simulink subsystem "Guidance_Team2"  (R2022b)
settings: Solver=VariableStepAuto  StartTime=0.0  StopTime=10.0  RelTol=1e-3
settings Model: Creator=Sahil Gaurkar  LastModifiedBy=Sahil Gaurkar

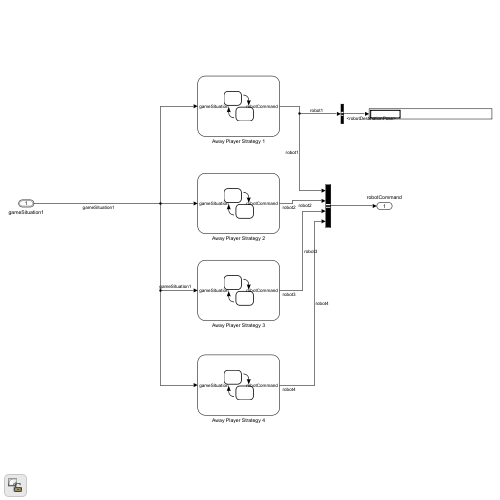
[thumbnail: Simulink's stored preview of the top-level diagram]
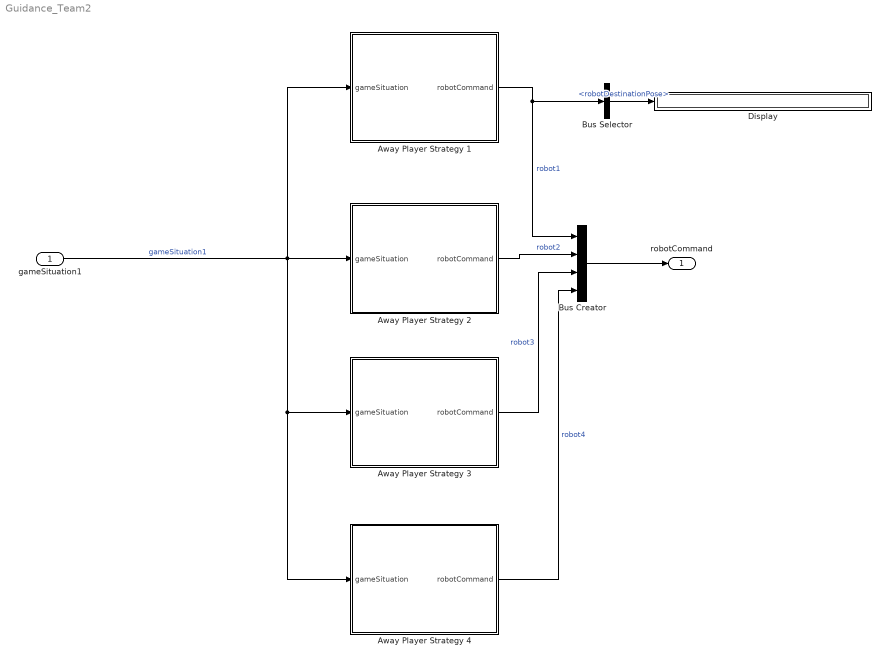
== system Guidance_Team2 ==
  gameSituation1 : Inport  OutDataTypeStr=Bus: gameSituation
  Away Player Strategy 1 : Stateflow chart  TreatAsAtomicUnit=on
  Away Player Strategy 2 : Stateflow chart  TreatAsAtomicUnit=on
  Away Player Strategy 3 : Stateflow chart  TreatAsAtomicUnit=on
  Away Player Strategy 4 : Stateflow chart  TreatAsAtomicUnit=on
  Bus Creator : BusCreator  Inputs=4
  Bus Selector : BusSelector  OutputSignals=robotDestinationPose
  Display : Display
  robotCommand : Outport
  wires:
  Away Player Strategy 3/1(robotCommand) -> Bus Creator/3  "robot3"
  gameSituation1/1 -> Away Player Strategy 3/1(gameSituation), Away Player Strategy 4/1(gameSituation), Away Player Strategy 1/1(gameSituation), Away Player Strategy 2/1(gameSituation)  "gameSituation1"
  Away Player Strategy 2/1(robotCommand) -> Bus Creator/2  "robot2"
  Bus Selector/1 -> Display/1  "<robotDestinationPose>"
  Away Player Strategy 4/1(robotCommand) -> Bus Creator/4  "robot4"
  Away Player Strategy 1/1(robotCommand) -> Bus Selector/1, Bus Creator/1  "robot1"
  Bus Creator/1 -> robotCommand/1

== stateflow chart Guidance_Team2/Away Player Strategy 1 ==
  state InitialState
    en,du:
    if gameSituation.kickConfirmation == true
    robotCommand.kick = false;
    end
    id = 1; % Team1(Home) Robot 1
    shootDistThres = 2500;
    kickableAreaRadius = 20;
    homeGoalPose = [5000, 0];
    awayGoalPose = [-5000, 0];
    homeAttackPositions = [[-3500, 0, 180]; [-2500, 1500, 180]; [-2500, -1500, 180]; [2500, 0, 180]];
    homeDefendPositions = [[1000, 0, 180]; [3000, 1500, 180]; [3000, -1500, 180]; [4000, 0, 180]];
  state ROBOT 1 [group]
    (Strategy for robot 1~3)
  state Attack
    en,du:
    %%calculate the distance to the goal
    teamDistToGoal = [0 0 0 0];
    for idx=1:1:4
    teamDistToGoal(idx) = distTo(gameSituation.robotCurrentPose(idx,1:2), awayGoalPose);
    end
    distToGoal1 = distTo(gameSituation.robotCurrentPose(id,1:2), awayGoalPose);
    %calculate the distance to the ball
    teamDistToBall = [0 0 0 0];
    for idx=1:1:4
    teamDistToBall(idx) = distTo(gameSituation.robotCurrentPose(idx,1:2), ...
    gameSituation.ballCurrentPose(1:2));
    end
    distToBall = distTo(gameSituation.robotCurrentPose(id,1:2), ...
    gameSituation.ballCurrentPose(1:2));
  state Defend
    en,du:
    %%calculate the distance to the home goal
    teamDistToOwnGoal = [0 0 0 0];
    for idx=1:1:4
    teamDistToOwnGoal(idx) = distTo(gameSituation.robotCurrentPose(idx,1:2), homeGoalPose);
    end
    distToOwnGoal = distTo(gameSituation.robotCurrentPose(id,1:2), homeGoalPose);
    for idx=1:1:4
    teamDistToBall(idx) = distTo(gameSituation.robotCurrentPose(idx,1:2), ...
    gameSituation.ballCurrentPose(1:2));
    end
    distToBall = distTo(gameSituation.robotCurrentPose(id,1:2), ...
    gameSituation.ballCurrentPose(1:2));
  state Position
    en,du:
    playerAttackPosition = homeAttackPositions(id, :);
    kickPower = 1;
    kickState = false;
    desiredPosition = playerAttackPosition;
    isdone = true;
  state Shoot
    en,du:
    angleBallGoal = atan2d(awayGoalPose(2) - gameSituation.ballCurrentPose(2), ...
    awayGoalPose(1) - gameSituation.ballCurrentPose(1));
    kickPower = 450;
    kickState = true;
    kickDirection = angleBallGoal;
    xPosition= gameSituation.ballCurrentPose(1) + cosd(180 - angleBallGoal) * kickableAreaRadius;
    yPosition = gameSituation.ballCurrentPose(2) + sind(180 - angleBallGoal) * kickableAreaRadius;
    desiredPosition = [xPosition, yPosition, kickDirection];
    isdone = true;
  state Pass
    en,du:
    [minval,minidx] = min(teamDistToGoal)
    angleBallPlayer = atan2d(gameSituation.robotCurrentPose(minidx, 2) - gameSituation.ballCurrentPose(2), ...
    gameSituation.robotCurrentPose(minidx, 1) - gameSituation.ballCurrentPose(1));
    distBallPlayer = norm(gameSituation.robotCurrentPose(minidx, 1:2) - gameSituation.ballCurrentPose(1:2));
    kickPower = distBallPlayer/4.9;
    kickState = true;
    kickDirection = angleBallPlayer;
    xPosition= gameSituation.ballCurrentPose(1) + cosd(180 - angleBallGoal) * kickableAreaRadius;
    yPosition = gameSituation.ballCurrentPose(2) + sind(180 - angleBallGoal) * kickableAreaRadius;
    desiredPosition = [xPosition, yPosition, kickDirection];
    isdone = true;
  state Dribble
    en,du:
    angleBallGoal = atan2d(awayGoalPose(2) - gameSituation.ballCurrentPose(2), ...
    awayGoalPose(1) - gameSituation.ballCurrentPose(1));
    kickPower = 100;
    %%should be designed as the kickPower = kickPowerCofficent * 100
    %%kickPowerCofficieant should also be calculated by distance
    kickState = true;
    kickDirection = angleBallGoal;
    xPosition= gameSituation.ballCurrentPose(1) + cosd(180 - angleBallGoal) * kickableAreaRadius;
    yPosition = gameSituation.ballCurrentPose(2) + sind(180 - angleBallGoal) * kickableAreaRadius;
    desiredPosition = [xPosition, yPosition, kickDirection];
    isdone = true;
  state Intercept
    en,du:
    angleBallGoal = gameSituation.robotCurrentPose(id, 3);
    kickPower = 150;
    kickState = true;
    kickDirection = angleBallGoal;
    xPosition= gameSituation.ballCurrentPose(1) + cosd(180 - angleBallGoal) * kickableAreaRadius;
    yPosition = gameSituation.ballCurrentPose(2) + sind(180 - angleBallGoal) * kickableAreaRadius;
    desiredPosition = [xPosition, yPosition, kickDirection];
    isdone = true;
  state Formation
    en,du:
    playerDefendPosition = homeDefendPositions(id, :);
    kickPower = 1;
    kickState = false;
    desiredPosition = playerDefendPosition;
    isdone = true;
  state Kick
    state MoveTo1
      en,du:
      isdone = false;
      robotCommand.robotDestinationPose = desiredPosition;
      distToBall = distTo(gameSituation.robotCurrentPose(id,1:2), ...
      gameSituation.ballCurrentPose(1:2));
    state KickTo
      en,du:
      robotCommand.kick = kickState;
      robotCommand.kickProperty = kickPower;
      isdone = true;
    MoveTo1 -> KickTo [order 1] : [distToBall <= kickableAreaRadius+5]
  MoveTo1 -> InitialState [order 2] : [after(1,sec)]
  KickTo -> InitialState : [after(1,sec)]
  (default) -> InitialState
  InitialState -> Attack [order 2] : [gameSituation.ballLastCommandBy(1) == 2]
  InitialState -> Defend [order 1] : [gameSituation.ballLastCommandBy(1) == 1]
  Attack -> Position [order 1] : [distToBall ~= min(teamDistToBall)]
  Defend -> Intercept [order 1] : [distToBall ~= max(teamDistToBall)]
  Defend -> Formation [order 2] : [distToBall == max(teamDistToBall)]
  Attack -> Pass [order 3] : [distToGoal1 ~= min(teamDistToGoal)&& distToBall == min(teamDistToBall)]
  Attack -> Dribble [order 4] : [distToBall == min(teamDistToBall) && distToGoal1 == min(teamDistToGoal) && distToGoal1 > shootDistThres]
  Attack -> Shoot [order 2] : [distToBall == min(teamDistToBall) && distToGoal1 == min(teamDistToGoal) && distToGoal1 < shootDistThres]
  Intercept -> MoveTo1 : [isdone]
  Formation -> MoveTo1 : [isdone]
  Pass -> MoveTo1 : [isdone]
  Dribble -> MoveTo1 : [isdone]
  Shoot -> MoveTo1 : [isdone]
  Position -> MoveTo1 : [isdone]
  data: robotPosition function_input; goalPosition function_input; dist function_output; awayGoalPose local =[0 0]; homeGoalPose local =[0 0]; id local =1; idx local; angleBallGoal local =0; desiredPosition local =[0 0 0]; distToOwnGoal local =0; kickDirection local =0; kickPower local =0; kickState local =false; minidx local; playerDefendPosition local =[0 0 0]; teamDistToGoal local =[0 0 0 0]; teamDistToOwnGoal local =[0 0 0 0]; minval local; isdone local boolean =false; playerAttackPosition local =[0 0 0]; shootDistThres local =0; gameSituation input Bus: gameSituation; kickableAreaRadius local =0; distToGoal1 local =0; angleBallPlayer local =0; robotCommand output Bus: robotCommand; distToBall local =0; teamDistToBall local =[0 0 0 0]; homeAttackPositions local =[0 0 0;0 0 0;0 0 0;0 0 0]; homeDefendPositions local =[0 0 0;0 0 0;0 0 0;0 0 0]; xPosition local; yPosition local; distBallPlayer local
  function dist = distTo(robotPosition,goalPosition):
    | function dist = distTo(robotPosition,goalPosition)
    |     dist = norm(robotPosition - goalPosition);
    | end

== stateflow chart Guidance_Team2/Away Player Strategy 2 ==
  state InitialState
    en,du:
    if gameSituation.kickConfirmation == true
    robotCommand.kick = false;
    end
    id = 2; % Team1(Home) Robot 1
    shootDistThres = 2500;
    kickableAreaRadius = 20;
    homeGoalPose = [5000, 0];
    awayGoalPose = [-5000, 0];
    homeAttackPositions = [[-3500, 0, 180]; [-2500, 1500, 180]; [-2500, -1500, 180]; [2500, 0, 180]];
    homeDefendPositions = [[1000, 0, 180]; [3000, 1500, 180]; [3000, -1500, 180]; [4000, 0, 180]];
  state ROBOT 1 [group]
    (Strategy for robot 1~3)
  state Attack
    en,du:
    %%calculate the distance to the goal
    teamDistToGoal = [0 0 0 0];
    for idx=1:1:4
    teamDistToGoal(idx) = distTo(gameSituation.robotCurrentPose(idx,1:2), awayGoalPose);
    end
    distToGoal1 = distTo(gameSituation.robotCurrentPose(id,1:2), awayGoalPose);
    %calculate the distance to the ball
    teamDistToBall = [0 0 0 0];
    for idx=1:1:4
    teamDistToBall(idx) = distTo(gameSituation.robotCurrentPose(idx,1:2), ...
    gameSituation.ballCurrentPose(1:2));
    end
    distToBall = distTo(gameSituation.robotCurrentPose(id,1:2), ...
    gameSituation.ballCurrentPose(1:2));
  state Defend
    en,du:
    %%calculate the distance to the home goal
    teamDistToOwnGoal = [0 0 0 0];
    for idx=1:1:4
    teamDistToOwnGoal(idx) = distTo(gameSituation.robotCurrentPose(idx,1:2), homeGoalPose);
    end
    distToOwnGoal = distTo(gameSituation.robotCurrentPose(id,1:2), homeGoalPose);
    for idx=1:1:4
    teamDistToBall(idx) = distTo(gameSituation.robotCurrentPose(idx,1:2), ...
    gameSituation.ballCurrentPose(1:2));
    end
    distToBall = distTo(gameSituation.robotCurrentPose(id,1:2), ...
    gameSituation.ballCurrentPose(1:2));
  state Position
    en,du:
    playerAttackPosition = homeAttackPositions(id, :);
    kickPower = 1;
    kickState = false;
    desiredPosition = playerAttackPosition;
    isdone = true;
  state Shoot
    en,du:
    angleBallGoal = atan2d(awayGoalPose(2) - gameSituation.ballCurrentPose(2), ...
    awayGoalPose(1) - gameSituation.ballCurrentPose(1));
    kickPower = 450;
    kickState = true;
    kickDirection = angleBallGoal;
    xPosition= gameSituation.ballCurrentPose(1) + cosd(180 - angleBallGoal) * kickableAreaRadius;
    yPosition = gameSituation.ballCurrentPose(2) + sind(180 - angleBallGoal) * kickableAreaRadius;
    desiredPosition = [xPosition, yPosition, kickDirection];
    isdone = true;
  state Pass
    en,du:
    [minval,minidx] = min(teamDistToGoal)
    angleBallPlayer = atan2d(gameSituation.robotCurrentPose(minidx, 2) - gameSituation.ballCurrentPose(2), ...
    gameSituation.robotCurrentPose(minidx, 1) - gameSituation.ballCurrentPose(1));
    distBallPlayer = norm(gameSituation.robotCurrentPose(minidx, 1:2) - gameSituation.ballCurrentPose(1:2));
    kickPower = distBallPlayer/4.9;
    kickState = true;
    kickDirection = angleBallPlayer;
    xPosition= gameSituation.ballCurrentPose(1) + cosd(180 - angleBallGoal) * kickableAreaRadius;
    yPosition = gameSituation.ballCurrentPose(2) + sind(180 - angleBallGoal) * kickableAreaRadius;
    desiredPosition = [xPosition, yPosition, kickDirection];
    isdone = true;
  state Dribble
    en,du:
    angleBallGoal = atan2d(awayGoalPose(2) - gameSituation.ballCurrentPose(2), ...
    awayGoalPose(1) - gameSituation.ballCurrentPose(1));
    kickPower = 100;
    %%should be designed as the kickPower = kickPowerCofficent * 100
    %%kickPowerCofficieant should also be calculated by distance
    kickState = true;
    kickDirection = angleBallGoal;
    xPosition= gameSituation.ballCurrentPose(1) + cosd(180 - angleBallGoal) * kickableAreaRadius;
    yPosition = gameSituation.ballCurrentPose(2) + sind(180 - angleBallGoal) * kickableAreaRadius;
    desiredPosition = [xPosition, yPosition, kickDirection];
    isdone = true;
  state Intercept
    en,du:
    angleBallGoal = gameSituation.robotCurrentPose(id, 3);
    kickPower = 150;
    kickState = true;
    kickDirection = angleBallGoal;
    xPosition= gameSituation.ballCurrentPose(1) + cosd(180 - angleBallGoal) * kickableAreaRadius;
    yPosition = gameSituation.ballCurrentPose(2) + sind(180 - angleBallGoal) * kickableAreaRadius;
    desiredPosition = [xPosition, yPosition, kickDirection];
    isdone = true;
  state Formation
    en,du:
    playerDefendPosition = homeDefendPositions(id, :);
    kickPower = 1;
    kickState = false;
    desiredPosition = playerDefendPosition;
    isdone = true;
  state Kick
    state MoveTo1
      en,du:
      isdone = false;
      robotCommand.robotDestinationPose = desiredPosition;
      distToBall = distTo(gameSituation.robotCurrentPose(id,1:2), ...
      gameSituation.ballCurrentPose(1:2));
    state KickTo
      en,du:
      robotCommand.kick = kickState;
      robotCommand.kickProperty = kickPower;
      isdone = true;
    MoveTo1 -> KickTo [order 1] : [distToBall <= kickableAreaRadius+5]
  MoveTo1 -> InitialState [order 2] : [after(1,sec)]
  KickTo -> InitialState : [after(1,sec)]
  (default) -> InitialState
  InitialState -> Attack [order 2] : [gameSituation.ballLastCommandBy(1) == 2]
  InitialState -> Defend [order 1] : [gameSituation.ballLastCommandBy(1) == 1]
  Attack -> Position [order 1] : [distToBall ~= min(teamDistToBall)]
  Defend -> Intercept [order 1] : [distToBall ~= max(teamDistToBall)]
  Defend -> Formation [order 2] : [distToBall == max(teamDistToBall)]
  Attack -> Pass [order 3] : [distToGoal1 ~= min(teamDistToGoal)&& distToBall == min(teamDistToBall)]
  Attack -> Dribble [order 4] : [distToBall == min(teamDistToBall) && distToGoal1 == min(teamDistToGoal) && distToGoal1 > shootDistThres]
  Attack -> Shoot [order 2] : [distToBall == min(teamDistToBall) && distToGoal1 == min(teamDistToGoal) && distToGoal1 < shootDistThres]
  Intercept -> MoveTo1 : [isdone]
  Formation -> MoveTo1 : [isdone]
  Pass -> MoveTo1 : [isdone]
  Dribble -> MoveTo1 : [isdone]
  Shoot -> MoveTo1 : [isdone]
  Position -> MoveTo1 : [isdone]
  data: robotPosition function_input; goalPosition function_input; dist function_output; awayGoalPose local =[0 0]; homeGoalPose local =[0 0]; id local =1; idx local; angleBallGoal local =0; desiredPosition local =[0 0 0]; distToOwnGoal local =0; kickDirection local =0; kickPower local =0; kickState local =false; minidx local; playerDefendPosition local =[0 0 0]; teamDistToGoal local =[0 0 0 0]; teamDistToOwnGoal local =[0 0 0 0]; minval local; isdone local boolean =false; playerAttackPosition local =[0 0 0]; shootDistThres local =0; gameSituation input Bus: gameSituation; kickableAreaRadius local =0; distToGoal1 local =0; angleBallPlayer local =0; robotCommand output Bus: robotCommand; distToBall local =0; teamDistToBall local =[0 0 0 0]; homeAttackPositions local =[0 0 0;0 0 0;0 0 0;0 0 0]; homeDefendPositions local =[0 0 0;0 0 0;0 0 0;0 0 0]; xPosition local; yPosition local; distBallPlayer local
  function dist = distTo(robotPosition,goalPosition):
    | function dist = distTo(robotPosition,goalPosition)
    |     dist = norm(robotPosition - goalPosition);
    | end

== stateflow chart Guidance_Team2/Away Player Strategy 3 ==
  state InitialState
    en,du:
    if gameSituation.kickConfirmation == true
    robotCommand.kick = false;
    end
    id = 3; % Team1(Home) Robot 1
    shootDistThres = 2500;
    kickableAreaRadius = 20;
    homeGoalPose = [5000, 0];
    awayGoalPose = [-5000, 0];
    homeAttackPositions = [[-3500, 0, 180]; [-2500, 1500, 180]; [-2500, -1500, 180]; [2500, 0, 180]];
    homeDefendPositions = [[1000, 0, 180]; [3000, 1500, 180]; [3000, -1500, 180]; [4000, 0, 180]];
  state ROBOT 1 [group]
    (Strategy for robot 1~3)
  state Attack
    en,du:
    %%calculate the distance to the goal
    teamDistToGoal = [0 0 0 0];
    for idx=1:1:4
    teamDistToGoal(idx) = distTo(gameSituation.robotCurrentPose(idx,1:2), awayGoalPose);
    end
    distToGoal1 = distTo(gameSituation.robotCurrentPose(id,1:2), awayGoalPose);
    %calculate the distance to the ball
    teamDistToBall = [0 0 0 0];
    for idx=1:1:4
    teamDistToBall(idx) = distTo(gameSituation.robotCurrentPose(idx,1:2), ...
    gameSituation.ballCurrentPose(1:2));
    end
    distToBall = distTo(gameSituation.robotCurrentPose(id,1:2), ...
    gameSituation.ballCurrentPose(1:2));
  state Defend
    en,du:
    %%calculate the distance to the home goal
    teamDistToOwnGoal = [0 0 0 0];
    for idx=1:1:4
    teamDistToOwnGoal(idx) = distTo(gameSituation.robotCurrentPose(idx,1:2), homeGoalPose);
    end
    distToOwnGoal = distTo(gameSituation.robotCurrentPose(id,1:2), homeGoalPose);
    for idx=1:1:4
    teamDistToBall(idx) = distTo(gameSituation.robotCurrentPose(idx,1:2), ...
    gameSituation.ballCurrentPose(1:2));
    end
    distToBall = distTo(gameSituation.robotCurrentPose(id,1:2), ...
    gameSituation.ballCurrentPose(1:2));
  state Position
    en,du:
    playerAttackPosition = homeAttackPositions(id, :);
    kickPower = 1;
    kickState = false;
    desiredPosition = playerAttackPosition;
    isdone = true;
  state Shoot
    en,du:
    angleBallGoal = atan2d(awayGoalPose(2) - gameSituation.ballCurrentPose(2), ...
    awayGoalPose(1) - gameSituation.ballCurrentPose(1));
    kickPower = 450;
    kickState = true;
    kickDirection = angleBallGoal;
    xPosition= gameSituation.ballCurrentPose(1) + cosd(180 - angleBallGoal) * kickableAreaRadius;
    yPosition = gameSituation.ballCurrentPose(2) + sind(180 - angleBallGoal) * kickableAreaRadius;
    desiredPosition = [xPosition, yPosition, kickDirection];
    isdone = true;
  state Pass
    en,du:
    [minval,minidx] = min(teamDistToGoal)
    angleBallPlayer = atan2d(gameSituation.robotCurrentPose(minidx, 2) - gameSituation.ballCurrentPose(2), ...
    gameSituation.robotCurrentPose(minidx, 1) - gameSituation.ballCurrentPose(1));
    distBallPlayer = norm(gameSituation.robotCurrentPose(minidx, 1:2) - gameSituation.ballCurrentPose(1:2));
    kickPower = distBallPlayer/4.9;
    kickState = true;
    kickDirection = angleBallPlayer;
    xPosition= gameSituation.ballCurrentPose(1) + cosd(180 - angleBallGoal) * kickableAreaRadius;
    yPosition = gameSituation.ballCurrentPose(2) + sind(180 - angleBallGoal) * kickableAreaRadius;
    desiredPosition = [xPosition, yPosition, kickDirection];
    isdone = true;
  state Dribble
    en,du:
    angleBallGoal = atan2d(awayGoalPose(2) - gameSituation.ballCurrentPose(2), ...
    awayGoalPose(1) - gameSituation.ballCurrentPose(1));
    kickPower = 100;
    %%should be designed as the kickPower = kickPowerCofficent * 100
    %%kickPowerCofficieant should also be calculated by distance
    kickState = true;
    kickDirection = angleBallGoal;
    xPosition= gameSituation.ballCurrentPose(1) + cosd(180 - angleBallGoal) * kickableAreaRadius;
    yPosition = gameSituation.ballCurrentPose(2) + sind(180 - angleBallGoal) * kickableAreaRadius;
    desiredPosition = [xPosition, yPosition, kickDirection];
    isdone = true;
  state Intercept
    en,du:
    angleBallGoal = gameSituation.robotCurrentPose(id, 3);
    kickPower = 150;
    kickState = true;
    kickDirection = angleBallGoal;
    xPosition= gameSituation.ballCurrentPose(1) + cosd(180 - angleBallGoal) * kickableAreaRadius;
    yPosition = gameSituation.ballCurrentPose(2) + sind(180 - angleBallGoal) * kickableAreaRadius;
    desiredPosition = [xPosition, yPosition, kickDirection];
    isdone = true;
  state Formation
    en,du:
    playerDefendPosition = homeDefendPositions(id, :);
    kickPower = 1;
    kickState = false;
    desiredPosition = playerDefendPosition;
    isdone = true;
  state Kick
    state MoveTo1
      en,du:
      isdone = false;
      robotCommand.robotDestinationPose = desiredPosition;
      distToBall = distTo(gameSituation.robotCurrentPose(id,1:2), ...
      gameSituation.ballCurrentPose(1:2));
    state KickTo
      en,du:
      robotCommand.kick = kickState;
      robotCommand.kickProperty = kickPower;
      isdone = true;
    MoveTo1 -> KickTo [order 1] : [distToBall <= kickableAreaRadius+5]
  MoveTo1 -> InitialState [order 2] : [after(1,sec)]
  KickTo -> InitialState : [after(1,sec)]
  (default) -> InitialState
  InitialState -> Attack [order 2] : [gameSituation.ballLastCommandBy(1) == 2]
  InitialState -> Defend [order 1] : [gameSituation.ballLastCommandBy(1) == 1]
  Attack -> Position [order 1] : [distToBall ~= min(teamDistToBall)]
  Defend -> Intercept [order 1] : [distToBall ~= max(teamDistToBall)]
  Defend -> Formation [order 2] : [distToBall == max(teamDistToBall)]
  Attack -> Pass [order 3] : [distToGoal1 ~= min(teamDistToGoal)&& distToBall == min(teamDistToBall)]
  Attack -> Dribble [order 4] : [distToBall == min(teamDistToBall) && distToGoal1 == min(teamDistToGoal) && distToGoal1 > shootDistThres]
  Attack -> Shoot [order 2] : [distToBall == min(teamDistToBall) && distToGoal1 == min(teamDistToGoal) && distToGoal1 < shootDistThres]
  Intercept -> MoveTo1 : [isdone]
  Formation -> MoveTo1 : [isdone]
  Pass -> MoveTo1 : [isdone]
  Dribble -> MoveTo1 : [isdone]
  Shoot -> MoveTo1 : [isdone]
  Position -> MoveTo1 : [isdone]
  data: robotPosition function_input; goalPosition function_input; dist function_output; awayGoalPose local =[0 0]; homeGoalPose local =[0 0]; id local =1; idx local; angleBallGoal local =0; desiredPosition local =[0 0 0]; distToOwnGoal local =0; kickDirection local =0; kickPower local =0; kickState local =false; minidx local; playerDefendPosition local =[0 0 0]; teamDistToGoal local =[0 0 0 0]; teamDistToOwnGoal local =[0 0 0 0]; minval local; isdone local boolean =false; playerAttackPosition local =[0 0 0]; shootDistThres local =0; gameSituation input Bus: gameSituation; kickableAreaRadius local =0; distToGoal1 local =0; angleBallPlayer local =0; robotCommand output Bus: robotCommand; distToBall local =0; teamDistToBall local =[0 0 0 0]; homeAttackPositions local =[0 0 0;0 0 0;0 0 0;0 0 0]; homeDefendPositions local =[0 0 0;0 0 0;0 0 0;0 0 0]; xPosition local; yPosition local; distBallPlayer local
  function dist = distTo(robotPosition,goalPosition):
    | function dist = distTo(robotPosition,goalPosition)
    |     dist = norm(robotPosition - goalPosition);
    | end

== stateflow chart Guidance_Team2/Away Player Strategy 4 ==
  state InitialState
    en,du:
    if gameSituation.kickConfirmation == true
    robotCommand.kick = false;
    end
    id = 4; % Team1(Home) Robot 1
    shootDistThres = 2500;
    kickableAreaRadius = 20;
    homeGoalPose = [5000, 0];
    awayGoalPose = [-5000, 0];
    homeAttackPositions = [[-3500, 0, 180]; [-2500, 1500, 180]; [-2500, -1500, 180]; [2500, 0, 180]];
    homeDefendPositions = [[1000, 0, 180]; [3000, 1500, 180]; [3000, -1500, 180]; [4000, 0, 180]];
  state ROBOT 1 [group]
    (Strategy for robot 1~3)
  state Attack
    en,du:
    %%calculate the distance to the goal
    teamDistToGoal = [0 0 0 0];
    for idx=1:1:4
    teamDistToGoal(idx) = distTo(gameSituation.robotCurrentPose(idx,1:2), awayGoalPose);
    end
    distToGoal1 = distTo(gameSituation.robotCurrentPose(id,1:2), awayGoalPose);
    %calculate the distance to the ball
    teamDistToBall = [0 0 0 0];
    for idx=1:1:4
    teamDistToBall(idx) = distTo(gameSituation.robotCurrentPose(idx,1:2), ...
    gameSituation.ballCurrentPose(1:2));
    end
    distToBall = distTo(gameSituation.robotCurrentPose(id,1:2), ...
    gameSituation.ballCurrentPose(1:2));
  state Defend
    en,du:
    %%calculate the distance to the home goal
    teamDistToOwnGoal = [0 0 0 0];
    for idx=1:1:4
    teamDistToOwnGoal(idx) = distTo(gameSituation.robotCurrentPose(idx,1:2), homeGoalPose);
    end
    distToOwnGoal = distTo(gameSituation.robotCurrentPose(id,1:2), homeGoalPose);
    for idx=1:1:4
    teamDistToBall(idx) = distTo(gameSituation.robotCurrentPose(idx,1:2), ...
    gameSituation.ballCurrentPose(1:2));
    end
    distToBall = distTo(gameSituation.robotCurrentPose(id,1:2), ...
    gameSituation.ballCurrentPose(1:2));
  state Position
    en,du:
    playerAttackPosition = homeAttackPositions(id, :);
    kickPower = 1;
    kickState = false;
    desiredPosition = playerAttackPosition;
    isdone = true;
  state Shoot
    en,du:
    angleBallGoal = atan2d(awayGoalPose(2) - gameSituation.ballCurrentPose(2), ...
    awayGoalPose(1) - gameSituation.ballCurrentPose(1));
    kickPower = 450;
    kickState = true;
    kickDirection = angleBallGoal;
    xPosition= gameSituation.ballCurrentPose(1) + cosd(180 - angleBallGoal) * kickableAreaRadius;
    yPosition = gameSituation.ballCurrentPose(2) + sind(180 - angleBallGoal) * kickableAreaRadius;
    desiredPosition = [xPosition, yPosition, kickDirection];
    isdone = true;
  state Pass
    en,du:
    [minval,minidx] = min(teamDistToGoal)
    angleBallPlayer = atan2d(gameSituation.robotCurrentPose(minidx, 2) - gameSituation.ballCurrentPose(2), ...
    gameSituation.robotCurrentPose(minidx, 1) - gameSituation.ballCurrentPose(1));
    distBallPlayer = norm(gameSituation.robotCurrentPose(minidx, 1:2) - gameSituation.ballCurrentPose(1:2));
    kickPower = distBallPlayer/4.9;
    kickState = true;
    kickDirection = angleBallPlayer;
    xPosition= gameSituation.ballCurrentPose(1) + cosd(180 - angleBallGoal) * kickableAreaRadius;
    yPosition = gameSituation.ballCurrentPose(2) + sind(180 - angleBallGoal) * kickableAreaRadius;
    desiredPosition = [xPosition, yPosition, kickDirection];
    isdone = true;
  state Dribble
    en,du:
    angleBallGoal = atan2d(awayGoalPose(2) - gameSituation.ballCurrentPose(2), ...
    awayGoalPose(1) - gameSituation.ballCurrentPose(1));
    kickPower = 100;
    %%should be designed as the kickPower = kickPowerCofficent * 100
    %%kickPowerCofficieant should also be calculated by distance
    kickState = true;
    kickDirection = angleBallGoal;
    xPosition= gameSituation.ballCurrentPose(1) + cosd(180 - angleBallGoal) * kickableAreaRadius;
    yPosition = gameSituation.ballCurrentPose(2) + sind(180 - angleBallGoal) * kickableAreaRadius;
    desiredPosition = [xPosition, yPosition, kickDirection];
    isdone = true;
  state Intercept
    en,du:
    angleBallGoal = gameSituation.robotCurrentPose(id, 3);
    kickPower = 150;
    kickState = true;
    kickDirection = angleBallGoal;
    xPosition= gameSituation.ballCurrentPose(1) + cosd(180 - angleBallGoal) * kickableAreaRadius;
    yPosition = gameSituation.ballCurrentPose(2) + sind(180 - angleBallGoal) * kickableAreaRadius;
    desiredPosition = [xPosition, yPosition, kickDirection];
    isdone = true;
  state Formation
    en,du:
    playerDefendPosition = homeDefendPositions(id, :);
    kickPower = 1;
    kickState = false;
    desiredPosition = playerDefendPosition;
    isdone = true;
  state Kick
    state MoveTo1
      en,du:
      isdone = false;
      robotCommand.robotDestinationPose = desiredPosition;
      distToBall = distTo(gameSituation.robotCurrentPose(id,1:2), ...
      gameSituation.ballCurrentPose(1:2));
    state KickTo
      en,du:
      robotCommand.kick = kickState;
      robotCommand.kickProperty = kickPower;
      isdone = true;
    MoveTo1 -> KickTo [order 1] : [distToBall <= kickableAreaRadius+5]
  MoveTo1 -> InitialState [order 2] : [after(1,sec)]
  KickTo -> InitialState : [after(1,sec)]
  (default) -> InitialState
  InitialState -> Attack [order 2] : [gameSituation.ballLastCommandBy(1) == 2]
  InitialState -> Defend [order 1] : [gameSituation.ballLastCommandBy(1) == 1]
  Attack -> Position [order 1] : [distToBall ~= min(teamDistToBall)]
  Defend -> Intercept [order 1] : [distToBall ~= max(teamDistToBall)]
  Defend -> Formation [order 2] : [distToBall == max(teamDistToBall)]
  Attack -> Pass [order 3] : [distToGoal1 ~= min(teamDistToGoal)&& distToBall == min(teamDistToBall)]
  Attack -> Dribble [order 4] : [distToBall == min(teamDistToBall) && distToGoal1 == min(teamDistToGoal) && distToGoal1 > shootDistThres]
  Attack -> Shoot [order 2] : [distToBall == min(teamDistToBall) && distToGoal1 == min(teamDistToGoal) && distToGoal1 < shootDistThres]
  Intercept -> MoveTo1 : [isdone]
  Formation -> MoveTo1 : [isdone]
  Pass -> MoveTo1 : [isdone]
  Dribble -> MoveTo1 : [isdone]
  Shoot -> MoveTo1 : [isdone]
  Position -> MoveTo1 : [isdone]
  data: robotPosition function_input; goalPosition function_input; dist function_output; awayGoalPose local =[0 0]; homeGoalPose local =[0 0]; id local =1; idx local; angleBallGoal local =0; desiredPosition local =[0 0 0]; distToOwnGoal local =0; kickDirection local =0; kickPower local =0; kickState local =false; minidx local; playerDefendPosition local =[0 0 0]; teamDistToGoal local =[0 0 0 0]; teamDistToOwnGoal local =[0 0 0 0]; minval local; isdone local boolean =false; playerAttackPosition local =[0 0 0]; shootDistThres local =0; gameSituation input Bus: gameSituation; kickableAreaRadius local =0; distToGoal1 local =0; angleBallPlayer local =0; robotCommand output Bus: robotCommand; distToBall local =0; teamDistToBall local =[0 0 0 0]; homeAttackPositions local =[0 0 0;0 0 0;0 0 0;0 0 0]; homeDefendPositions local =[0 0 0;0 0 0;0 0 0;0 0 0]; xPosition local; yPosition local; distBallPlayer local
  function dist = distTo(robotPosition,goalPosition):
    | function dist = distTo(robotPosition,goalPosition)
    |     dist = norm(robotPosition - goalPosition);
    | end
